simulink model "BMS"  (R2021a)
settings: Solver=VariableStepAuto  StartTime=0.0  StopTime=3600  RelTol=1e-3
settings Model: Creator=mohandes  LastModifiedBy=mohandes

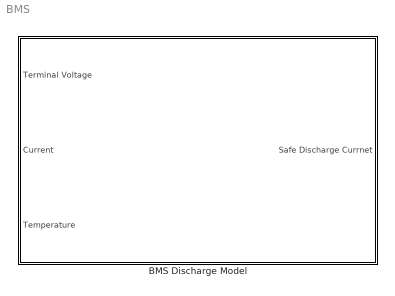
== system BMS ==
  BMS Discharge Model : Subsystem
      mask Display: image('F:\Gen-Hub Academy\Round 1\Simulink\EV\BMS\Photos\BMS.jpg'); % Use "Edit Image" on toolstrip to change.

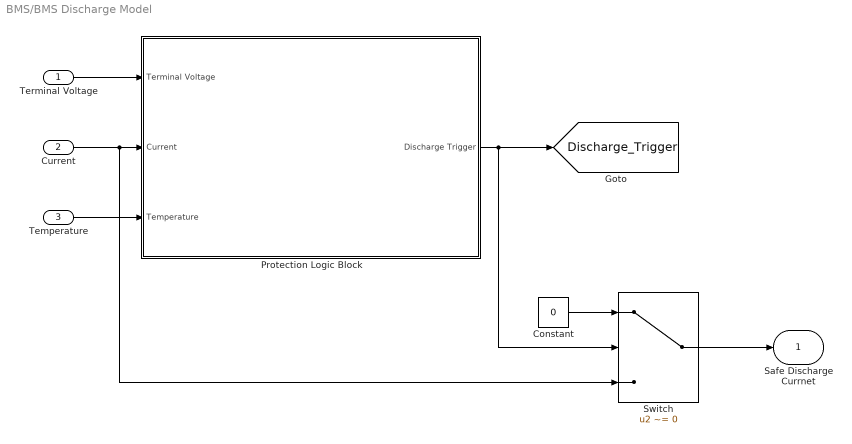
== system BMS/BMS Discharge Model ==
  Terminal Voltage : Inport
  Current : Inport  Port=2
  Temperature : Inport  Port=3
  Constant : Constant  Value=0
  Protection Logic Block : Subsystem
      mask Display: image('F:\Gen-Hub Academy\Round 1\Simulink\EV\BMS\Photos\Protection.jpg'); % Use "Edit Image" on toolstrip to change.
  Switch : Switch  Criteria=u2 ~= 0
  Safe Discharge Currnet : Outport
  tag scope: Discharge_Trigger=global
  wires:
  Terminal Voltage/1 -> Protection Logic Block/1(Terminal Voltage)
  Current/1 -> Switch/3, Protection Logic Block/2(Current)
  Temperature/1 -> Protection Logic Block/3(Temperature)
  Protection Logic Block/1(Discharge Trigger) -> Switch/2, [Discharge_Trigger]
  Constant/1 -> Switch/1
  Switch/1 -> Safe Discharge Currnet/1

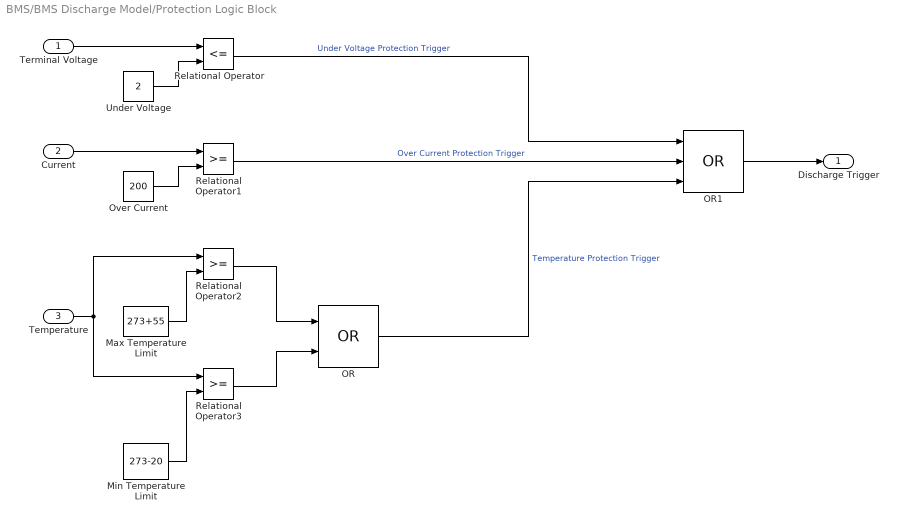
== system BMS/BMS Discharge Model/Protection Logic Block ==
  Terminal Voltage : Inport
  Current : Inport  Port=2
  Temperature : Inport  Port=3
  Max Temperature Limit : Constant  Value=273+55
  Min Temperature Limit : Constant  Value=273-20
  OR : Logic  Operator=OR  IconShape=distinctive  AllPortsSameDT=off  OutDataTypeStr=boolean
  OR1 : Logic  Operator=OR  Inputs=3  IconShape=distinctive  AllPortsSameDT=off  OutDataTypeStr=boolean
  Over Current : Constant  Value=200
  Relational Operator : RelationalOperator  Operator=<=  OutDataTypeStr=boolean  RndMeth=Simplest
  Relational Operator1 : RelationalOperator  OutDataTypeStr=boolean  RndMeth=Simplest
  Relational Operator2 : RelationalOperator  OutDataTypeStr=boolean  RndMeth=Simplest
  Relational Operator3 : RelationalOperator  OutDataTypeStr=boolean  RndMeth=Simplest
  Under Voltage : Constant  Value=2
  Discharge Trigger : Outport
  wires:
  Under Voltage/1 -> Relational Operator/2
  Terminal Voltage/1 -> Relational Operator/1
  Current/1 -> Relational Operator1/1
  Over Current/1 -> Relational Operator1/2
  Temperature/1 -> Relational Operator3/1, Relational Operator2/1
  Max Temperature Limit/1 -> Relational Operator2/2
  Min Temperature Limit/1 -> Relational Operator3/2
  Relational Operator2/1 -> OR/1
  Relational Operator3/1 -> OR/2
  OR1/1 -> Discharge Trigger/1
  OR/1 -> OR1/3  "Temperature Protection Trigger"
  Relational Operator1/1 -> OR1/2  "Over Current Protection Trigger"
  Relational Operator/1 -> OR1/1  "Under Voltage Protection Trigger"
